simulink model "tank"  (R2018b)
settings: Solver=VariableStepAuto  StartTime=0.0  StopTime=240  RelTol=1e-3
settings Model: Creator=kjartan  LastModifiedBy=kjartan

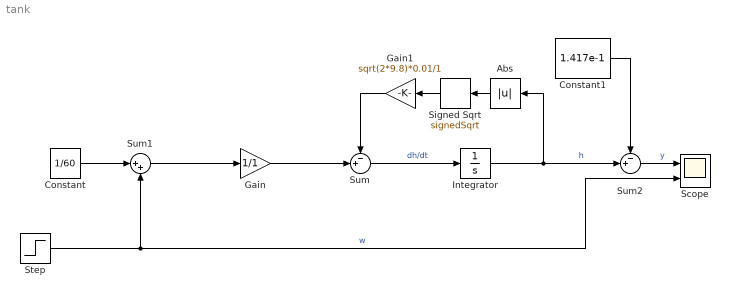
== system tank ==
  Abs : Abs
  Constant : Constant  Value=1/60
  Constant1 : Constant  Value=1.417e-1
  Gain : Gain  Gain=1/1
  Gain1 : Gain  Gain=sqrt(2*9.8)*0.01/1
  Integrator : Integrator  InitialCondition=(1/60)*(1/60)/0.01/0.01/2/9.8
  Scope : Scope  NumInputPorts=2
  Signed Sqrt : Sqrt  Operator=signedSqrt  SaturateOnIntegerOverflow=on
  Step : Step  Time=10  After=3/60  SampleTime=0
  Sum : Sum  Inputs=-+|
  Sum1 : Sum  Inputs=|++
  Sum2 : Sum  Inputs=-+|
  wires:
  Integrator/1 -> Sum2/2, Abs/1  "h"
  Sum/1 -> Integrator/1  "dh/dt"
  Sum1/1 -> Gain/1
  Gain/1 -> Sum/2
  Abs/1 -> Signed Sqrt/1
  Signed Sqrt/1 -> Gain1/1
  Gain1/1 -> Sum/1
  Step/1 -> Scope/2, Sum1/2  "w"
  Constant/1 -> Sum1/1
  Constant1/1 -> Sum2/1
  Sum2/1 -> Scope/1  "y"
